simulink model "FOC_PIL_top_"  (R2020b)
settings: Solver=FixedStepAuto  StartTime=0.0  StopTime=4  FixedStep=Ts  RelTol=1e-3
undefined symbols (not defined in the file or in its folder): motor
libraries: mcbplantlib x1, autolibpmsminterior x1
settings Model: Creator=k  LastModifiedBy=k

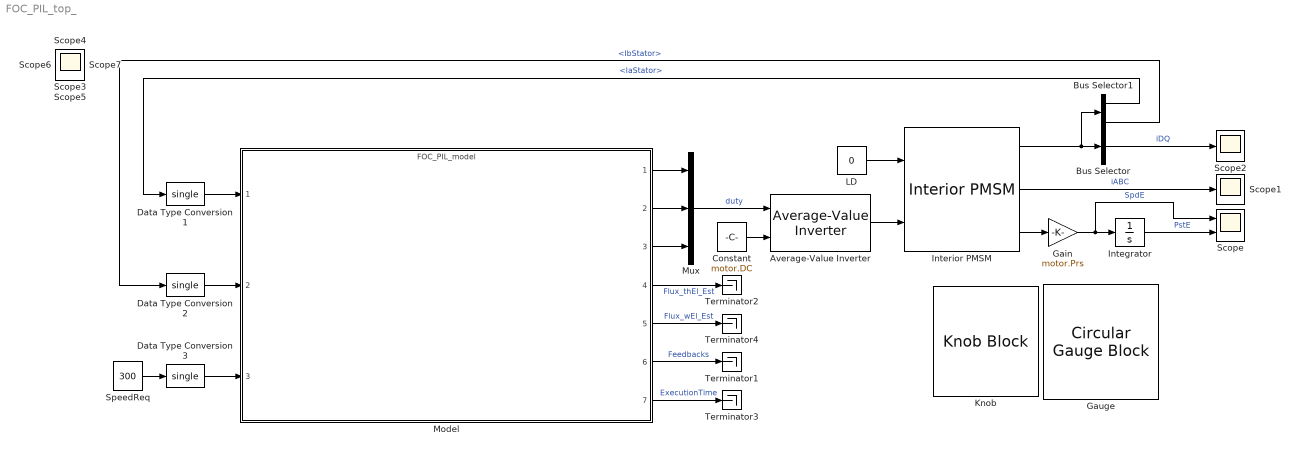
== system FOC_PIL_top_ ==
  Average-Value Inverter : mcbplantlib/Average-Value Inverter
  Bus Selector : BusSelector  OutputSignals=IdSync,IqSync  OutputAsBus=on
  Bus Selector1 : BusSelector  OutputSignals=IaStator,IbStator
  Constant : Constant  Value=motor.DC
  Data Type Conversion1 : DataTypeConversion  OutDataTypeStr=single
  Data Type Conversion2 : DataTypeConversion  OutDataTypeStr=single
  Data Type Conversion3 : DataTypeConversion  OutDataTypeStr=single
  Gain : Gain  Gain=motor.Prs
  Gauge : CircularGaugeBlock  ScaleMin=-3.14  ScaleMax=3.14  TickInterval=1.57
  Integrator : Integrator  WrapState=on  WrappedStateUpperValue=2*pi  WrappedStateLowerValue=0
  Interior PMSM : autolibpmsminterior/Interior PMSM  port_config=Torque  sim_type=Continuous  Ts=0.001  P=motor.Prs  Rs=motor.Rs  Ldq=[motor.Ld motor.Lq]  KConstText=Permanent flux linkage constant (lambda_pm):  lambda_pm=motor.Flux  Ke=159.9771  mechanical=[motor.J, motor.B, motor.Tf]  idq0=[0 0]  theta_init=0  omega_init=0  KConst=motor.Flux  lambda_pm_calc=motor.Flux  Kt=0.07  RefBlkName='autolibpmsminterior/Interior PMSM'  aMode=5
      settings: SourceProductBaseCode=PW,MT,UV,VE,VP
  Knob : KnobBlock  ScaleMin=100  ScaleMax=400
  LD : Constant  Value=0
  Model : ModelReference  ModelNameDialog=FOC_PIL_model.slx  SimulationMode=Processor-in-the-loop (PIL)  ModelReferenceVersion=1.582
  Mux : Mux  Inputs=3
  Scope : Scope  NumInputPorts=2
  Scope{1..7} (7 alike) : Scope
  SpeedReq : Constant  Value=300
  Terminator{1..4} (4 alike) : Terminator
  wires:
  Integrator/1 -> Scope/2  "PstE"
  Model/3 -> Mux/3
  Bus Selector/1 -> Scope2/1  "iDQ"
  LD/1 -> Interior PMSM/1
  Interior PMSM/1 -> Bus Selector1/1, Bus Selector/1
  Bus Selector1/1 -> Data Type Conversion1/1  "<IaStator>"
  Model/2 -> Mux/2
  Gain/1 -> Integrator/1, Scope/1  "SpdE"
  Interior PMSM/2 -> Scope1/1  "iABC"
  Bus Selector1/2 -> Data Type Conversion2/1  "<IbStator>"
  Model/1 -> Mux/1
  Interior PMSM/3 -> Gain/1
  Mux/1 -> Average-Value Inverter/1  "duty"
  Average-Value Inverter/1 -> Interior PMSM/2
  Constant/1 -> Average-Value Inverter/2
  Data Type Conversion1/1 -> Model/1
  Data Type Conversion2/1 -> Model/2
  Model/4 -> Terminator2/1  "Flux_thEl_Est"
  Model/7 -> Terminator3/1  "ExecutionTime"
  Model/5 -> Terminator4/1  "Flux_wEl_Est"
  Model/6 -> Terminator1/1  "Feedbacks"
  Data Type Conversion3/1 -> Model/3
  SpeedReq/1 -> Data Type Conversion3/1
